simulink model "Dnote3lv3rd"  (R2016b)
settings: Solver=FixedStepDiscrete  StartTime=0.0  StopTime=simtime  RelTol=1e-3  EnableMultiTasking=on
PreLoadFcn:
  | simtime=0.0034;
undefined symbols (not defined in the file): Amp, fdesignblkfcn, Fin, Fs, FSC, gcbh, N, p, sw1, Ts
libraries: simulink x153, dspsnks4 x2, dspfdesign x1, dspvision x1, dsparch4 x1, dspmlti4 x1
(part 3 of 3)

== system Dnote3lv3rd/3-level NSDEM /P_SELECTOR/Subsystem7 ==
  In1 : Inport
  Combinatorial Logic : CombinatorialLogic  TruthTable=[0 0 0 0 0 0 0 0;1 0 0 0 0 0 0 0]
  Combinatorial Logic1 : CombinatorialLogic  TruthTable=[0 0 0 0 0 0 0 0; 0 1 0 0 0 0 0 0]
  Combinatorial Logic2 : CombinatorialLogic  TruthTable=[0 0 0 0 0 0 0 0;0 0 1 0 0 0 0 0]
  Combinatorial Logic3 : CombinatorialLogic  TruthTable=[0 0 0 0 0 0 0 0;0 0 0 1 0 0 0 0]
  Combinatorial Logic4 : CombinatorialLogic  TruthTable=[0 0 0 0 0 0 0 0;0 0 0 0 1 0 0 0]
  Combinatorial Logic5 : CombinatorialLogic  TruthTable=[0 0 0 0 0 0 0 0;0 0 0 0 0 1 0 0]
  Combinatorial Logic6 : CombinatorialLogic  TruthTable=[0 0 0 0 0 0 0 0;0 0 0 0 0 0 1 0]
  Combinatorial Logic7 : CombinatorialLogic  TruthTable=[0 0 0 0 0 0 0 0;0 0 0 0 0 0 0 1]
  Compare To Constnt : simulink/Logic and Bit Operations/Compare To Constant  relop===  const=0  OutDataTypeStr=boolean  ZeroCross=off
  Compare To Constnt1 : simulink/Logic and Bit Operations/Compare To Constant  relop===  const=1  OutDataTypeStr=boolean  ZeroCross=off
  Compare To Constnt2 : simulink/Logic and Bit Operations/Compare To Constant  relop===  const=2  OutDataTypeStr=boolean  ZeroCross=off
  Compare To Constnt3 : simulink/Logic and Bit Operations/Compare To Constant  relop===  const=3  OutDataTypeStr=boolean  ZeroCross=off
  Compare To Constnt4 : simulink/Logic and Bit Operations/Compare To Constant  relop===  const=4  OutDataTypeStr=boolean  ZeroCross=off
  Compare To Constnt5 : simulink/Logic and Bit Operations/Compare To Constant  relop===  const=5  OutDataTypeStr=boolean  ZeroCross=off
  Compare To Constnt6 : simulink/Logic and Bit Operations/Compare To Constant  relop===  const=6  OutDataTypeStr=boolean  ZeroCross=off
  Compare To Constnt7 : simulink/Logic and Bit Operations/Compare To Constant  relop===  const=7  OutDataTypeStr=boolean  ZeroCross=off
  Logical Operator : Logic  Operator=OR  Inputs=8  AllPortsSameDT=off  OutDataTypeStr=boolean
  Out1 : Outport
  wires:
  Logical Operator/1 -> Out1/1
  In1/1 -> Compare To Constnt5/1, Compare To Constnt6/1, Compare To Constnt7/1, Compare To Constnt4/1, Compare To Constnt3/1, Compare To Constnt2/1, Compare To Constnt1/1, Compare To Constnt/1
  Compare To Constnt/1 -> Combinatorial Logic/1
  Compare To Constnt1/1 -> Combinatorial Logic1/1
  Compare To Constnt2/1 -> Combinatorial Logic2/1
  Compare To Constnt3/1 -> Combinatorial Logic3/1
  Compare To Constnt4/1 -> Combinatorial Logic4/1
  Compare To Constnt5/1 -> Combinatorial Logic5/1
  Compare To Constnt6/1 -> Combinatorial Logic6/1
  Compare To Constnt7/1 -> Combinatorial Logic7/1
  Combinatorial Logic/1 -> Logical Operator/1
  Combinatorial Logic1/1 -> Logical Operator/2
  Combinatorial Logic2/1 -> Logical Operator/3
  Combinatorial Logic3/1 -> Logical Operator/4
  Combinatorial Logic4/1 -> Logical Operator/5
  Combinatorial Logic5/1 -> Logical Operator/6
  Combinatorial Logic6/1 -> Logical Operator/7
  Combinatorial Logic7/1 -> Logical Operator/8

== system Dnote3lv3rd/3-level NSDEM /Sort16/XSW ==
  IP : Inport
  IM : Inport  Port=2
  SP : Inport  Port=3
  SM : Inport  Port=4
  Relational Operator : RelationalOperator  Operator=<  OutDataTypeStr=boolean  RndMeth=Nearest
  Switch{,1..3} (4 alike) : Switch  Criteria=u2 > Threshold
  OA : Outport
  OB : Outport  Port=2
  QA : Outport  Port=3
  QB : Outport  Port=4
  wires:
  Switch3/1 -> QB/1
  Switch2/1 -> QA/1
  SM/1 -> Switch2/3, Switch3/1
  SP/1 -> Switch2/1, Switch3/3
  Switch1/1 -> OB/1
  Switch/1 -> OA/1
  Relational Operator/1 -> Switch3/2, Switch2/2, Switch1/2, Switch/2
  IM/1 -> Switch/3, Switch1/1, Relational Operator/2
  IP/1 -> Switch1/3, Switch/1, Relational Operator/1

== system Dnote3lv3rd/3-level NSDEM /Sort16/XSW1 ==
  IM : Inport
  IP : Inport  Port=2
  SM : Inport  Port=3
  SP : Inport  Port=4
  Relational Operator : RelationalOperator  Operator=<  OutDataTypeStr=boolean  RndMeth=Nearest
  Switch{,1..3} (4 alike) : Switch  Criteria=u2 > Threshold
  OB : Outport
  OA : Outport  Port=2
  QB : Outport  Port=3
  QA : Outport  Port=4
  wires:
  IP/1 -> Relational Operator/1, Switch/1, Switch1/3
  IM/1 -> Relational Operator/2, Switch1/1, Switch/3
  Relational Operator/1 -> Switch/2, Switch1/2, Switch2/2, Switch3/2
  Switch/1 -> OA/1
  Switch1/1 -> OB/1
  SP/1 -> Switch3/3, Switch2/1
  SM/1 -> Switch3/1, Switch2/3
  Switch2/1 -> QA/1
  Switch3/1 -> QB/1

== system Dnote3lv3rd/3-level NSDEM /Sort16/XSW10 ==
  IM : Inport
  IP : Inport  Port=2
  SM : Inport  Port=3
  SP : Inport  Port=4
  Relational Operator : RelationalOperator  Operator=<  OutDataTypeStr=boolean  RndMeth=Nearest
  Switch{,1..3} (4 alike) : Switch  Criteria=u2 > Threshold
  OB : Outport
  OA : Outport  Port=2
  QB : Outport  Port=3
  QA : Outport  Port=4
  wires:
  IP/1 -> Relational Operator/1, Switch/1, Switch1/3
  IM/1 -> Relational Operator/2, Switch1/1, Switch/3
  Relational Operator/1 -> Switch/2, Switch1/2, Switch2/2, Switch3/2
  Switch/1 -> OA/1
  Switch1/1 -> OB/1
  SP/1 -> Switch3/3, Switch2/1
  SM/1 -> Switch3/1, Switch2/3
  Switch2/1 -> QA/1
  Switch3/1 -> QB/1

== system Dnote3lv3rd/3-level NSDEM /Sort16/XSW11 ==
  IM : Inport
  IP : Inport  Port=2
  SM : Inport  Port=3
  SP : Inport  Port=4
  Relational Operator : RelationalOperator  Operator=<  OutDataTypeStr=boolean  RndMeth=Nearest
  Switch{,1..3} (4 alike) : Switch  Criteria=u2 > Threshold
  OB : Outport
  OA : Outport  Port=2
  QB : Outport  Port=3
  QA : Outport  Port=4
  wires:
  Switch3/1 -> QB/1
  Switch2/1 -> QA/1
  SM/1 -> Switch2/3, Switch3/1
  SP/1 -> Switch2/1, Switch3/3
  Switch1/1 -> OB/1
  Switch/1 -> OA/1
  Relational Operator/1 -> Switch3/2, Switch2/2, Switch1/2, Switch/2
  IM/1 -> Switch/3, Switch1/1, Relational Operator/2
  IP/1 -> Switch1/3, Switch/1, Relational Operator/1

== system Dnote3lv3rd/3-level NSDEM /Sort16/XSW12 ==
  IP : Inport
  IM : Inport  Port=2
  SP : Inport  Port=3
  SM : Inport  Port=4
  Relational Operator : RelationalOperator  Operator=<  OutDataTypeStr=boolean  RndMeth=Nearest
  Switch{,1..3} (4 alike) : Switch  Criteria=u2 > Threshold
  OA : Outport
  OB : Outport  Port=2
  QA : Outport  Port=3
  QB : Outport  Port=4
  wires:
  Switch3/1 -> QB/1
  Switch2/1 -> QA/1
  SM/1 -> Switch2/3, Switch3/1
  SP/1 -> Switch2/1, Switch3/3
  Switch1/1 -> OB/1
  Switch/1 -> OA/1
  Relational Operator/1 -> Switch3/2, Switch2/2, Switch1/2, Switch/2
  IM/1 -> Switch/3, Switch1/1, Relational Operator/2
  IP/1 -> Switch1/3, Switch/1, Relational Operator/1

== system Dnote3lv3rd/3-level NSDEM /Sort16/XSW13 ==
  IP : Inport
  IM : Inport  Port=2
  SP : Inport  Port=3
  SM : Inport  Port=4
  Relational Operator : RelationalOperator  Operator=<  OutDataTypeStr=boolean  RndMeth=Nearest
  Switch{,1..3} (4 alike) : Switch  Criteria=u2 > Threshold
  OA : Outport
  OB : Outport  Port=2
  QA : Outport  Port=3
  QB : Outport  Port=4
  wires:
  IP/1 -> Relational Operator/1, Switch/1, Switch1/3
  IM/1 -> Relational Operator/2, Switch1/1, Switch/3
  Relational Operator/1 -> Switch/2, Switch1/2, Switch2/2, Switch3/2
  Switch/1 -> OA/1
  Switch1/1 -> OB/1
  SP/1 -> Switch3/3, Switch2/1
  SM/1 -> Switch3/1, Switch2/3
  Switch2/1 -> QA/1
  Switch3/1 -> QB/1

== system Dnote3lv3rd/3-level NSDEM /Sort16/XSW14 ==
  IP : Inport
  IM : Inport  Port=2
  SP : Inport  Port=3
  SM : Inport  Port=4
  Relational Operator : RelationalOperator  Operator=<  OutDataTypeStr=boolean  RndMeth=Nearest
  Switch{,1..3} (4 alike) : Switch  Criteria=u2 > Threshold
  OA : Outport
  OB : Outport  Port=2
  QA : Outport  Port=3
  QB : Outport  Port=4
  wires:
  Switch3/1 -> QB/1
  Switch2/1 -> QA/1
  SM/1 -> Switch2/3, Switch3/1
  SP/1 -> Switch2/1, Switch3/3
  Switch1/1 -> OB/1
  Switch/1 -> OA/1
  Relational Operator/1 -> Switch3/2, Switch2/2, Switch1/2, Switch/2
  IM/1 -> Switch/3, Switch1/1, Relational Operator/2
  IP/1 -> Switch1/3, Switch/1, Relational Operator/1

== system Dnote3lv3rd/3-level NSDEM /Sort16/XSW15 ==
  IP : Inport
  IM : Inport  Port=2
  SP : Inport  Port=3
  SM : Inport  Port=4
  Relational Operator : RelationalOperator  Operator=<  OutDataTypeStr=boolean  RndMeth=Nearest
  Switch{,1..3} (4 alike) : Switch  Criteria=u2 > Threshold
  OA : Outport
  OB : Outport  Port=2
  QA : Outport  Port=3
  QB : Outport  Port=4
  wires:
  IP/1 -> Relational Operator/1, Switch/1, Switch1/3
  IM/1 -> Relational Operator/2, Switch1/1, Switch/3
  Relational Operator/1 -> Switch/2, Switch1/2, Switch2/2, Switch3/2
  Switch/1 -> OA/1
  Switch1/1 -> OB/1
  SP/1 -> Switch3/3, Switch2/1
  SM/1 -> Switch3/1, Switch2/3
  Switch2/1 -> QA/1
  Switch3/1 -> QB/1

== system Dnote3lv3rd/3-level NSDEM /Sort16/XSW16 ==
  IP : Inport
  IM : Inport  Port=2
  SP : Inport  Port=3
  SM : Inport  Port=4
  Relational Operator : RelationalOperator  Operator=<  OutDataTypeStr=boolean  RndMeth=Nearest
  Switch{,1..3} (4 alike) : Switch  Criteria=u2 > Threshold
  OA : Outport
  OB : Outport  Port=2
  QA : Outport  Port=3
  QB : Outport  Port=4
  wires:
  IP/1 -> Relational Operator/1, Switch/1, Switch1/3
  IM/1 -> Relational Operator/2, Switch1/1, Switch/3
  Relational Operator/1 -> Switch/2, Switch1/2, Switch2/2, Switch3/2
  Switch/1 -> OA/1
  Switch1/1 -> OB/1
  SP/1 -> Switch3/3, Switch2/1
  SM/1 -> Switch3/1, Switch2/3
  Switch2/1 -> QA/1
  Switch3/1 -> QB/1

== system Dnote3lv3rd/3-level NSDEM /Sort16/XSW17 ==
  IP : Inport
  IM : Inport  Port=2
  SP : Inport  Port=3
  SM : Inport  Port=4
  Relational Operator : RelationalOperator  Operator=<  OutDataTypeStr=boolean  RndMeth=Nearest
  Switch{,1..3} (4 alike) : Switch  Criteria=u2 > Threshold
  OA : Outport
  OB : Outport  Port=2
  QA : Outport  Port=3
  QB : Outport  Port=4
  wires:
  Switch3/1 -> QB/1
  Switch2/1 -> QA/1
  SM/1 -> Switch2/3, Switch3/1
  SP/1 -> Switch2/1, Switch3/3
  Switch1/1 -> OB/1
  Switch/1 -> OA/1
  Relational Operator/1 -> Switch3/2, Switch2/2, Switch1/2, Switch/2
  IM/1 -> Switch/3, Switch1/1, Relational Operator/2
  IP/1 -> Switch1/3, Switch/1, Relational Operator/1

== system Dnote3lv3rd/3-level NSDEM /Sort16/XSW18 ==
  IP : Inport
  IM : Inport  Port=2
  SP : Inport  Port=3
  SM : Inport  Port=4
  Relational Operator : RelationalOperator  Operator=<  OutDataTypeStr=boolean  RndMeth=Nearest
  Switch{,1..3} (4 alike) : Switch  Criteria=u2 > Threshold
  OA : Outport
  OB : Outport  Port=2
  QA : Outport  Port=3
  QB : Outport  Port=4
  wires:
  IP/1 -> Relational Operator/1, Switch/1, Switch1/3
  IM/1 -> Relational Operator/2, Switch1/1, Switch/3
  Relational Operator/1 -> Switch/2, Switch1/2, Switch2/2, Switch3/2
  Switch/1 -> OA/1
  Switch1/1 -> OB/1
  SP/1 -> Switch3/3, Switch2/1
  SM/1 -> Switch3/1, Switch2/3
  Switch2/1 -> QA/1
  Switch3/1 -> QB/1

== system Dnote3lv3rd/3-level NSDEM /Sort16/XSW19 ==
  IP : Inport
  IM : Inport  Port=2
  SP : Inport  Port=3
  SM : Inport  Port=4
  Relational Operator : RelationalOperator  Operator=<  OutDataTypeStr=boolean  RndMeth=Nearest
  Switch{,1..3} (4 alike) : Switch  Criteria=u2 > Threshold
  OA : Outport
  OB : Outport  Port=2
  QA : Outport  Port=3
  QB : Outport  Port=4
  wires:
  Switch3/1 -> QB/1
  Switch2/1 -> QA/1
  SM/1 -> Switch2/3, Switch3/1
  SP/1 -> Switch2/1, Switch3/3
  Switch1/1 -> OB/1
  Switch/1 -> OA/1
  Relational Operator/1 -> Switch3/2, Switch2/2, Switch1/2, Switch/2
  IM/1 -> Switch/3, Switch1/1, Relational Operator/2
  IP/1 -> Switch1/3, Switch/1, Relational Operator/1

== system Dnote3lv3rd/3-level NSDEM /Sort16/XSW2 ==
  IP : Inport
  IM : Inport  Port=2
  SP : Inport  Port=3
  SM : Inport  Port=4
  Relational Operator : RelationalOperator  Operator=<  OutDataTypeStr=boolean  RndMeth=Nearest
  Switch{,1..3} (4 alike) : Switch  Criteria=u2 > Threshold
  OA : Outport
  OB : Outport  Port=2
  QA : Outport  Port=3
  QB : Outport  Port=4
  wires:
  IP/1 -> Relational Operator/1, Switch/1, Switch1/3
  IM/1 -> Relational Operator/2, Switch1/1, Switch/3
  Relational Operator/1 -> Switch/2, Switch1/2, Switch2/2, Switch3/2
  Switch/1 -> OA/1
  Switch1/1 -> OB/1
  SP/1 -> Switch3/3, Switch2/1
  SM/1 -> Switch3/1, Switch2/3
  Switch2/1 -> QA/1
  Switch3/1 -> QB/1

== system Dnote3lv3rd/3-level NSDEM /Sort16/XSW20 ==
  IP : Inport
  IM : Inport  Port=2
  SP : Inport  Port=3
  SM : Inport  Port=4
  Relational Operator : RelationalOperator  Operator=<  OutDataTypeStr=boolean  RndMeth=Nearest
  Switch{,1..3} (4 alike) : Switch  Criteria=u2 > Threshold
  OA : Outport
  OB : Outport  Port=2
  QA : Outport  Port=3
  QB : Outport  Port=4
  wires:
  IP/1 -> Relational Operator/1, Switch/1, Switch1/3
  IM/1 -> Relational Operator/2, Switch1/1, Switch/3
  Relational Operator/1 -> Switch/2, Switch1/2, Switch2/2, Switch3/2
  Switch/1 -> OA/1
  Switch1/1 -> OB/1
  SP/1 -> Switch3/3, Switch2/1
  SM/1 -> Switch3/1, Switch2/3
  Switch2/1 -> QA/1
  Switch3/1 -> QB/1

== system Dnote3lv3rd/3-level NSDEM /Sort16/XSW21 ==
  IP : Inport
  IM : Inport  Port=2
  SP : Inport  Port=3
  SM : Inport  Port=4
  Relational Operator : RelationalOperator  Operator=<  OutDataTypeStr=boolean  RndMeth=Nearest
  Switch{,1..3} (4 alike) : Switch  Criteria=u2 > Threshold
  OA : Outport
  OB : Outport  Port=2
  QA : Outport  Port=3
  QB : Outport  Port=4
  wires:
  Switch3/1 -> QB/1
  Switch2/1 -> QA/1
  SM/1 -> Switch2/3, Switch3/1
  SP/1 -> Switch2/1, Switch3/3
  Switch1/1 -> OB/1
  Switch/1 -> OA/1
  Relational Operator/1 -> Switch3/2, Switch2/2, Switch1/2, Switch/2
  IM/1 -> Switch/3, Switch1/1, Relational Operator/2
  IP/1 -> Switch1/3, Switch/1, Relational Operator/1

== system Dnote3lv3rd/3-level NSDEM /Sort16/XSW22 ==
  IP : Inport
  IM : Inport  Port=2
  SP : Inport  Port=3
  SM : Inport  Port=4
  Relational Operator : RelationalOperator  Operator=<  OutDataTypeStr=boolean  RndMeth=Nearest
  Switch{,1..3} (4 alike) : Switch  Criteria=u2 > Threshold
  OA : Outport
  OB : Outport  Port=2
  QA : Outport  Port=3
  QB : Outport  Port=4
  wires:
  Switch3/1 -> QB/1
  Switch2/1 -> QA/1
  SM/1 -> Switch2/3, Switch3/1
  SP/1 -> Switch2/1, Switch3/3
  Switch1/1 -> OB/1
  Switch/1 -> OA/1
  Relational Operator/1 -> Switch3/2, Switch2/2, Switch1/2, Switch/2
  IM/1 -> Switch/3, Switch1/1, Relational Operator/2
  IP/1 -> Switch1/3, Switch/1, Relational Operator/1

== system Dnote3lv3rd/3-level NSDEM /Sort16/XSW23 ==
  IP : Inport
  IM : Inport  Port=2
  SP : Inport  Port=3
  SM : Inport  Port=4
  Relational Operator : RelationalOperator  Operator=<  OutDataTypeStr=boolean  RndMeth=Nearest
  Switch{,1..3} (4 alike) : Switch  Criteria=u2 > Threshold
  OA : Outport
  OB : Outport  Port=2
  QA : Outport  Port=3
  QB : Outport  Port=4
  wires:
  IP/1 -> Relational Operator/1, Switch/1, Switch1/3
  IM/1 -> Relational Operator/2, Switch1/1, Switch/3
  Relational Operator/1 -> Switch/2, Switch1/2, Switch2/2, Switch3/2
  Switch/1 -> OA/1
  Switch1/1 -> OB/1
  SP/1 -> Switch3/3, Switch2/1
  SM/1 -> Switch3/1, Switch2/3
  Switch2/1 -> QA/1
  Switch3/1 -> QB/1

== system Dnote3lv3rd/3-level NSDEM /Sort16/XSW3 ==
  IM : Inport
  IP : Inport  Port=2
  SM : Inport  Port=3
  SP : Inport  Port=4
  Relational Operator : RelationalOperator  Operator=<  OutDataTypeStr=boolean  RndMeth=Nearest
  Switch{,1..3} (4 alike) : Switch  Criteria=u2 > Threshold
  OB : Outport
  OA : Outport  Port=2
  QB : Outport  Port=3
  QA : Outport  Port=4
  wires:
  Switch3/1 -> QB/1
  Switch2/1 -> QA/1
  SM/1 -> Switch2/3, Switch3/1
  SP/1 -> Switch2/1, Switch3/3
  Switch1/1 -> OB/1
  Switch/1 -> OA/1
  Relational Operator/1 -> Switch3/2, Switch2/2, Switch1/2, Switch/2
  IM/1 -> Switch/3, Switch1/1, Relational Operator/2
  IP/1 -> Switch1/3, Switch/1, Relational Operator/1

== system Dnote3lv3rd/3-level NSDEM /Sort16/XSW4 ==
  IP : Inport
  IM : Inport  Port=2
  SP : Inport  Port=3
  SM : Inport  Port=4
  Relational Operator : RelationalOperator  Operator=<  OutDataTypeStr=boolean  RndMeth=Nearest
  Switch{,1..3} (4 alike) : Switch  Criteria=u2 > Threshold
  OA : Outport
  OB : Outport  Port=2
  QA : Outport  Port=3
  QB : Outport  Port=4
  wires:
  IP/1 -> Relational Operator/1, Switch/1, Switch1/3
  IM/1 -> Relational Operator/2, Switch1/1, Switch/3
  Relational Operator/1 -> Switch/2, Switch1/2, Switch2/2, Switch3/2
  Switch/1 -> OA/1
  Switch1/1 -> OB/1
  SP/1 -> Switch3/3, Switch2/1
  SM/1 -> Switch3/1, Switch2/3
  Switch2/1 -> QA/1
  Switch3/1 -> QB/1

== system Dnote3lv3rd/3-level NSDEM /Sort16/XSW5 ==
  IP : Inport
  IM : Inport  Port=2
  SP : Inport  Port=3
  SM : Inport  Port=4
  Relational Operator : RelationalOperator  Operator=<  OutDataTypeStr=boolean  RndMeth=Nearest
  Switch{,1..3} (4 alike) : Switch  Criteria=u2 > Threshold
  OA : Outport
  OB : Outport  Port=2
  QA : Outport  Port=3
  QB : Outport  Port=4
  wires:
  Switch3/1 -> QB/1
  Switch2/1 -> QA/1
  SM/1 -> Switch2/3, Switch3/1
  SP/1 -> Switch2/1, Switch3/3
  Switch1/1 -> OB/1
  Switch/1 -> OA/1
  Relational Operator/1 -> Switch3/2, Switch2/2, Switch1/2, Switch/2
  IM/1 -> Switch/3, Switch1/1, Relational Operator/2
  IP/1 -> Switch1/3, Switch/1, Relational Operator/1

== system Dnote3lv3rd/3-level NSDEM /Sort16/XSW6 ==
  IM : Inport
  IP : Inport  Port=2
  SM : Inport  Port=3
  SP : Inport  Port=4
  Relational Operator : RelationalOperator  Operator=<  OutDataTypeStr=boolean  RndMeth=Nearest
  Switch{,1..3} (4 alike) : Switch  Criteria=u2 > Threshold
  OB : Outport
  OA : Outport  Port=2
  QB : Outport  Port=3
  QA : Outport  Port=4
  wires:
  Switch3/1 -> QB/1
  Switch2/1 -> QA/1
  SM/1 -> Switch2/3, Switch3/1
  SP/1 -> Switch2/1, Switch3/3
  Switch1/1 -> OB/1
  Switch/1 -> OA/1
  Relational Operator/1 -> Switch3/2, Switch2/2, Switch1/2, Switch/2
  IM/1 -> Switch/3, Switch1/1, Relational Operator/2
  IP/1 -> Switch1/3, Switch/1, Relational Operator/1

== system Dnote3lv3rd/3-level NSDEM /Sort16/XSW7 ==
  IM : Inport
  IP : Inport  Port=2
  SM : Inport  Port=3
  SP : Inport  Port=4
  Relational Operator : RelationalOperator  Operator=<  OutDataTypeStr=boolean  RndMeth=Nearest
  Switch{,1..3} (4 alike) : Switch  Criteria=u2 > Threshold
  OB : Outport
  OA : Outport  Port=2
  QB : Outport  Port=3
  QA : Outport  Port=4
  wires:
  IP/1 -> Relational Operator/1, Switch/1, Switch1/3
  IM/1 -> Relational Operator/2, Switch1/1, Switch/3
  Relational Operator/1 -> Switch/2, Switch1/2, Switch2/2, Switch3/2
  Switch/1 -> OA/1
  Switch1/1 -> OB/1
  SP/1 -> Switch3/3, Switch2/1
  SM/1 -> Switch3/1, Switch2/3
  Switch2/1 -> QA/1
  Switch3/1 -> QB/1

== system Dnote3lv3rd/3-level NSDEM /Sort16/XSW8 ==
  IP : Inport
  IM : Inport  Port=2
  SP : Inport  Port=3
  SM : Inport  Port=4
  Relational Operator : RelationalOperator  Operator=<  OutDataTypeStr=boolean  RndMeth=Nearest
  Switch{,1..3} (4 alike) : Switch  Criteria=u2 > Threshold
  OA : Outport
  OB : Outport  Port=2
  QA : Outport  Port=3
  QB : Outport  Port=4
  wires:
  Switch3/1 -> QB/1
  Switch2/1 -> QA/1
  SM/1 -> Switch2/3, Switch3/1
  SP/1 -> Switch2/1, Switch3/3
  Switch1/1 -> OB/1
  Switch/1 -> OA/1
  Relational Operator/1 -> Switch3/2, Switch2/2, Switch1/2, Switch/2
  IM/1 -> Switch/3, Switch1/1, Relational Operator/2
  IP/1 -> Switch1/3, Switch/1, Relational Operator/1

== system Dnote3lv3rd/3-level NSDEM /Sort16/XSW9 ==
  IP : Inport
  IM : Inport  Port=2
  SP : Inport  Port=3
  SM : Inport  Port=4
  Relational Operator : RelationalOperator  Operator=<  OutDataTypeStr=boolean  RndMeth=Nearest
  Switch{,1..3} (4 alike) : Switch  Criteria=u2 > Threshold
  OA : Outport
  OB : Outport  Port=2
  QA : Outport  Port=3
  QB : Outport  Port=4
  wires:
  IP/1 -> Relational Operator/1, Switch/1, Switch1/3
  IM/1 -> Relational Operator/2, Switch1/1, Switch/3
  Relational Operator/1 -> Switch/2, Switch1/2, Switch2/2, Switch3/2
  Switch/1 -> OA/1
  Switch1/1 -> OB/1
  SP/1 -> Switch3/3, Switch2/1
  SM/1 -> Switch3/1, Switch2/3
  Switch2/1 -> QA/1
  Switch3/1 -> QB/1
